simulink model "using_matlab_inverse_kinematics"  (R2021a)
settings: Solver=VariableStepAuto  StartTime=0.0  StopTime=10.0  RelTol=1e-3
values from neighbouring files (symbols this model uses):
  s = servo(a, 'D9', 'MinPulseDuration', 700e-6, 'MaxPulseDuration', 2300e-6)    [Untitled.m]
undefined symbols (not defined in the file or in its folder): smiData, X, Y, Z
libraries: sm_lib x146, nesl_utility x13
(part 1 of 4)
settings Model: Creator=user  LastModifiedBy=user

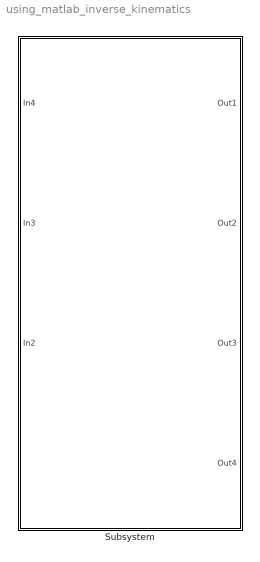
== system using_matlab_inverse_kinematics ==
  Subsystem : Subsystem
